simulink model "QuarterCarModel"  (R2018b)
settings: Solver=VariableStepAuto  StartTime=0.0  StopTime=10.0  RelTol=1e-3
values from neighbouring files (symbols this model uses):
  cs_c = 1000    [parameters.m]
  cs_e = cs_c    (= 1000)    [parameters.m]
  g = 9.81    [parameters.m]
  ks = 2e4    (= 20000)    [parameters.m]
  kstiff = ks    (= 20000)    [parameters.m]
  kt = 14e4    (= 140000)    [parameters.m]
  m1 = 250    [parameters.m]
  m2 = 20    [parameters.m]
  x0 = 0.2    [parameters.m]
settings Model: Creator=Hannah  LastModifiedBy=Hannah

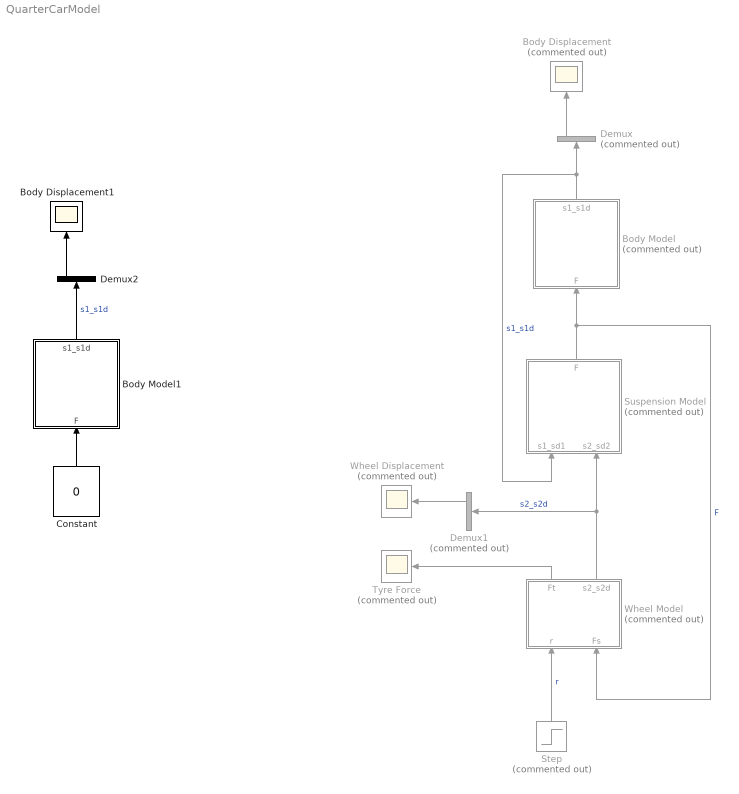
== system QuarterCarModel ==
  Body Displacement : Scope  Commented=on
  Body Displacement1 : Scope
  Body Model : Subsystem  Commented=on
  Body Model1 : Subsystem
  Constant : Constant  Value=0
  Demux : Demux  Commented=on  Outputs=2
  Demux1 : Demux  Commented=on  Outputs=2
  Demux2 : Demux  Outputs=2
  Step : Step  Commented=on  SampleTime=0
  Suspension Model : Subsystem  Commented=on
  Tyre Force : Scope  Commented=on
  Wheel Displacement : Scope  Commented=on
  Wheel Model : Subsystem  Commented=on
  wires:
  Body Model/1(s1_s1d) -> Demux/1, Suspension Model/1(s1_sd1)  "s1_s1d"
  Suspension Model/1(F) -> Wheel Model/2(Fs), Body Model/1(F)  "F"
  Wheel Model/2(s2_s2d) -> Demux1/1, Suspension Model/2(s2_sd2)  "s2_s2d"
  Step/1 -> Wheel Model/1(r)  "r"
  Demux/1 -> Body Displacement/1
  Demux1/1 -> Wheel Displacement/1
  Wheel Model/1(Ft) -> Tyre Force/1
  Body Model1/1(s1_s1d) -> Demux2/1  "s1_s1d"
  Demux2/1 -> Body Displacement1/1
  Constant/1 -> Body Model1/1(F)

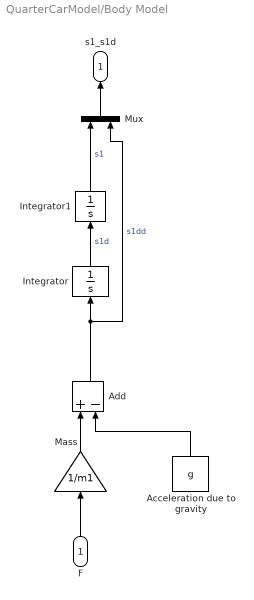
== system QuarterCarModel/Body Model ==
  F : Inport
  "Acceleration due to gravity " : Constant  Value=g
  Add : Sum  Inputs=+-
  Integrator : Integrator
  Integrator1 : Integrator
  Mass : Gain  Gain=1/m1
  Mux : Mux  Inputs=2
  s1_s1d : Outport
  wires:
  Mux/1 -> s1_s1d/1
  Mass/1 -> Add/1
  Integrator/1 -> Integrator1/1  "s1d"
  "Acceleration due to gravity "/1 -> Add/2
  F/1 -> Mass/1
  Integrator1/1 -> Mux/1  "s1"
  Add/1 -> Mux/2, Integrator/1  "s1dd"

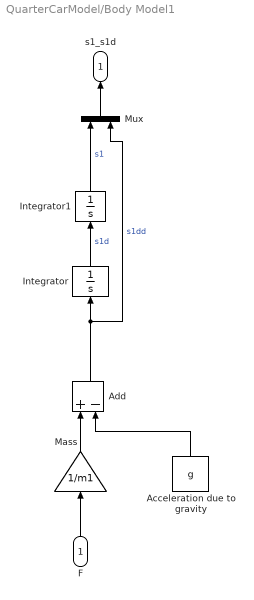
== system QuarterCarModel/Body Model1 ==
  F : Inport
  "Acceleration due to gravity " : Constant  Value=g
  Add : Sum  Inputs=+-
  Integrator : Integrator
  Integrator1 : Integrator
  Mass : Gain  Gain=1/m1
  Mux : Mux  Inputs=2
  s1_s1d : Outport
  wires:
  Mux/1 -> s1_s1d/1
  Mass/1 -> Add/1
  Integrator/1 -> Integrator1/1  "s1d"
  "Acceleration due to gravity "/1 -> Add/2
  F/1 -> Mass/1
  Integrator1/1 -> Mux/1  "s1"
  Add/1 -> Mux/2, Integrator/1  "s1dd"

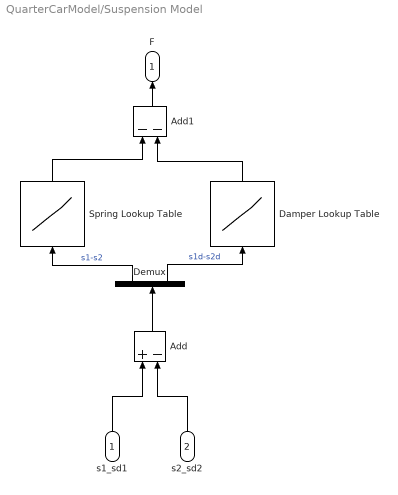
== system QuarterCarModel/Suspension Model ==
  s1_sd1 : Inport
  s2_sd2 : Inport  Port=2
  Add : Sum  Inputs=+-
  Add1 : Sum  Inputs=--
  Damper Lookup Table : Lookup_n-D  NumberOfTableDimensions=1  BreakpointsForDimension1=[-1 0 1]  Table=[-cs_c, 0, cs_e]  InternalRulePriority=Speed  RndMeth=Simplest  InputSameDT=on
  Demux : Demux  Outputs=2
  Spring Lookup Table : Lookup_n-D  NumberOfTableDimensions=1  BreakpointsForDimension1=[-2*x0, -x0, x0, 2*x0]  Table=[-(ks+kstiff)*x0, -ks*x0, ks*x0, (ks+kstiff)*x0]  InternalRulePriority=Speed  RndMeth=Simplest  InputSameDT=on
  F : Outport
  wires:
  s2_sd2/1 -> Add/2
  Spring Lookup Table/1 -> Add1/1
  Add1/1 -> F/1
  Damper Lookup Table/1 -> Add1/2
  Demux/2 -> Damper Lookup Table/1  "s1d-s2d"
  Demux/1 -> Spring Lookup Table/1  "s1-s2"
  Add/1 -> Demux/1
  s1_sd1/1 -> Add/1

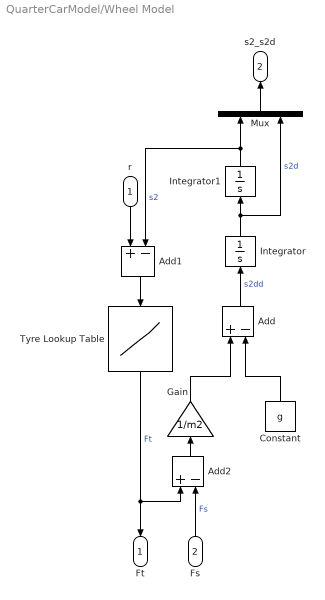
== system QuarterCarModel/Wheel Model ==
  r : Inport
  Fs : Inport  Port=2
  Add : Sum  Inputs=+-
  Add1 : Sum  Inputs=+-
  Add2 : Sum  Inputs=+-
  Constant : Constant  Value=g
  Gain : Gain  Gain=1/m2
  Integrator : Integrator
  Integrator1 : Integrator
  Mux : Mux  Inputs=2
  Tyre Lookup Table : Lookup_n-D  NumberOfTableDimensions=1  BreakpointsForDimension1=[-1 0 1]  Table=[0, 0, kt]  InternalRulePriority=Speed  RndMeth=Simplest  InputSameDT=on
  Ft : Outport
  s2_s2d : Outport  Port=2
  wires:
  r/1 -> Add1/1
  Fs/1 -> Add2/2  "Fs"
  Add2/1 -> Gain/1
  Gain/1 -> Add/1
  Integrator/1 -> Mux/2, Integrator1/1  "s2d"
  Add/1 -> Integrator/1  "s2dd"
  Tyre Lookup Table/1 -> Ft/1, Add2/1  "Ft"
  Constant/1 -> Add/2
  Integrator1/1 -> Add1/2, Mux/1  "s2"
  Add1/1 -> Tyre Lookup Table/1
  Mux/1 -> s2_s2d/1
